simulink model "prac221"  (R2022b)
settings: Solver=VariableStepAuto  StartTime=0.0  StopTime=100  RelTol=1e-3
settings Model: Creator=ESTHER  LastModifiedBy=ESTHER

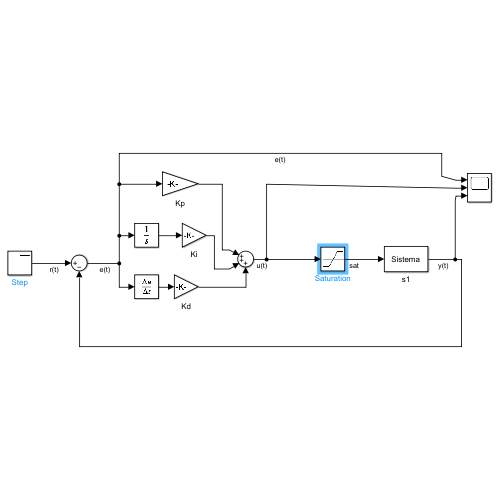
[thumbnail: Simulink's stored preview of the top-level diagram]
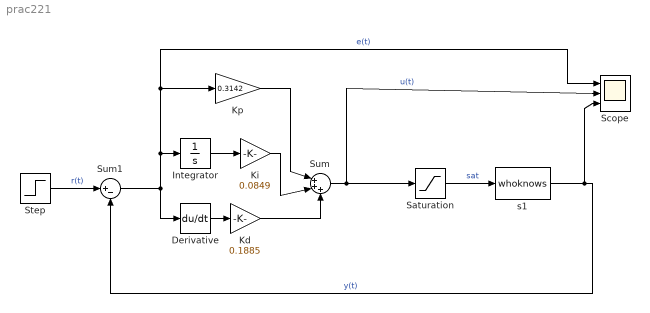
== system prac221 ==
  Derivative : Derivative
  Integrator : Integrator
  Kd : Gain  Gain=0.1885
  Ki : Gain  Gain=0.0849
  Kp : Gain  Gain=0.3142
  Saturation : Saturate  UpperLimit=3.2e+05  LowerLimit=-8.1e+04
  Scope : Scope  NumInputPorts=3
  Step : Step  SampleTime=0
  Sum : Sum  Inputs=|+++
  Sum1 : Sum  Inputs=|+-
  s1 : M-S-Function  FunctionName=whoknows  Parameters=L, P1, P2, T, R  mask{L=6, P1=1, P2=3, T=1, R=0}
      mask prompts: L "Laboratorio"; P1 "Primer digito del Puesto"; P2 "Segundo digito del Puesto"; T "Tipo de Planta"; R "Ruido"
      mask Display: disp('Sistema')
  wires:
  s1/1 -> Scope/3, Sum1/2  "y(t)"
  Sum/1 -> Saturation/1, Scope/2  "u(t)"
  Step/1 -> Sum1/1  "r(t)"
  Sum1/1 -> Integrator/1, Scope/1, Kp/1, Derivative/1  "e(t)"
  Derivative/1 -> Kd/1
  Integrator/1 -> Ki/1
  Kp/1 -> Sum/1
  Ki/1 -> Sum/2
  Kd/1 -> Sum/3
  Saturation/1 -> s1/1  "sat"
